simulink model "3_inverse_dynamics_TL"  (R2019b)
settings: Solver=VariableStepAuto  StartTime=0.0  StopTime=2  RelTol=1e-3
undefined symbols (not defined in the file or in its folder): DiscIntNeverNeededParam
libraries: powerlib x4, powerlib_extras x2, simulink x2
settings Model: Creator=liuzhong  LastModifiedBy=李瑾年
settings SFSimCC: CustomCodeUndefinedFunction=UseInterfaceOnly

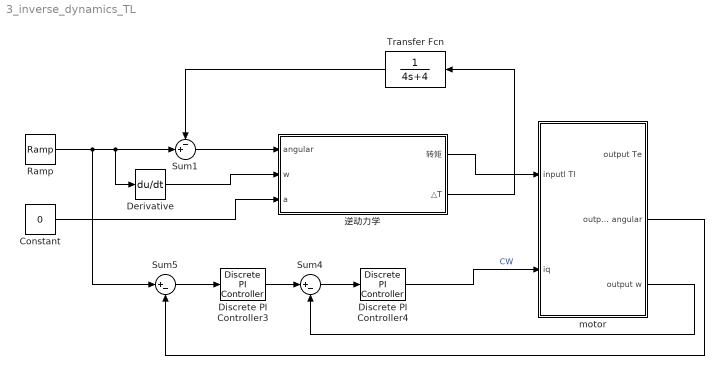
== system 3_inverse_dynamics_TL ==
  Constant : Constant  Value=0
  Derivative : Derivative
  Discrete PI Controller3 : powerlib_extras/Discrete  Control Blocks/Discrete PI Controller  Kp=140  Ki=90  Par_Limits=[1000 -1000]  Init=0  Ts=50e-6
      settings: SourceProductName=Simscape Electrical
  Discrete PI Controller4 : powerlib_extras/Discrete  Control Blocks/Discrete PI Controller  Kp=0.01897  Ki=1.9986  Par_Limits=[300 -300]  Init=0  Ts=50e-6
      settings: SourceProductName=Simscape Electrical
  Ramp : simulink/Sources/Ramp  slope=pi  start=0  InitialOutput=0
  Sum1 : Sum  Inputs=-+|
  Sum4 : Sum  Inputs=|+-
  Sum5 : Sum  Inputs=|+-
  Transfer Fcn : TransferFcn  Denominator=[4 4]
  motor : Subsystem
  逆动力学 : Subsystem
  wires:
  逆动力学/1(转矩) -> motor/1(inputl Tl)
  Sum4/1 -> Discrete PI Controller4/1
  Discrete PI Controller3/1 -> Sum4/1
  Sum5/1 -> Discrete PI Controller3/1
  motor/2(output angular) -> Sum5/2
  motor/3(output w) -> Sum4/2
  Discrete PI Controller4/1 -> motor/2("iq ")  "CW"
  Ramp/1 -> Sum5/1, Sum1/2, Derivative/1
  Derivative/1 -> 逆动力学/2(w)
  Constant/1 -> 逆动力学/3(a)
  逆动力学/2(△T) -> Transfer Fcn/1
  Sum1/1 -> 逆动力学/1("angular ")
  Transfer Fcn/1 -> Sum1/1

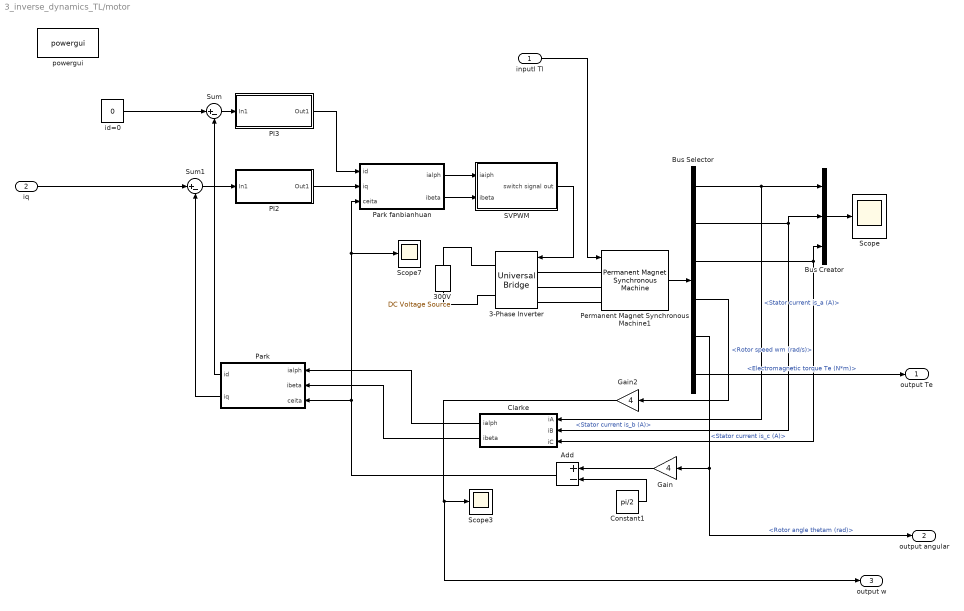
== system 3_inverse_dynamics_TL/motor ==
  inputl Tl : Inport
  "iq " : Inport  Port=2
  3-Phase Inverter : powerlib/Power Electronics/Universal Bridge  Arms=3  SnubberResistance=1e5  SnubberCapacitance=inf  Device=IGBT / Diodes  Ron=1e-3  Lon=0  ForwardVoltages="[  0  0  ]"  ForwardVoltage=0  GTOparameters=[ 10e-6 , 20e-6 ]  IGBTparameters=[ 1e-6 , 2e-6 ]  Measurements=None  Measurements_2=None  converterType=Rectifier
      settings: SourceProductName=Simscape Electrical
  300V : powerlib/Electrical Sources/DC Voltage Source  Amplitude=300  Measurements=Voltage
      settings: SourceProductName=Simscape Electrical
  Add : Sum  Inputs=+-
  Bus Creator : BusCreator  Inputs=3
  Bus Selector : BusSelector  OutputSignals=Stator current is_a (A),Stator current is_b (A),Stator current is_c (A),Rotor speed wm (rad/s),Rotor angle thetam (rad),Electromagnetic torque Te (N*m)
  Clarke : Subsystem
  Constant1 : Constant  Value=pi/2
  Gain : Gain  Gain=4
  Gain2 : Gain  Gain=4
  PI2 : Subsystem
  PI3 : Subsystem
  Park : Subsystem
  Park fanbianhuan : Subsystem
  Permanent Magnet Synchronous Machine1 : powerlib/Machines/Permanent Magnet Synchronous Machine  NbPhases=3  FluxDistribution=Sinusoidal  RotorType=Round  MechanicalLoad=Torque Tm  PresetModel=No  ShowDetailedParameters=on  MeasurementBus=off  Resistance=0.901  Inductance=8.5e-3  dqInductances=[0.02682 0.02682]  La=0.006365  MachineConstant=Torque Constant (N.m / A_peak)  Flux=0.13333  VoltageCst=96.736  TorqueCst=0.8  Flat=120  Mechanical=[0.00012 0.0008 4]  PolePairs=2  InitialConditions=[0,0, 0,0]  InitialConditions5ph=[0 0 0 0 0 0]  RefAngle=90 degrees behind phase A axis (modified Park)  IterativeDiscreteModel=Trapezoidal non iterative  TsBlock=-1  TsPowergui=0
  SVPWM : Subsystem
  Scope : Scope
  Scope3 : Scope
  Scope7 : Scope
  Sum : Sum  Inputs=|+-
  Sum1 : Sum  Inputs=|+-
  id=0 : Constant  Value=0
  powergui : powerlib/powergui  Priority=1  SimulationMode=Discrete  SampleTime=1e-6  frequency=60  Iterations=50  frequencyindice=0  Pbase=100e6  ErrMax=1e-4  UnitsV=kV  UnitsW=MW  buscounter=0  FunctionMessages=off  echomessages=off  EnableUseOfTLC=off  CurrentSourceSwitches=off  DisableSnubberDevices=off  DisableRonSwitches=off  DisableVfSwitches=off  DisplayEquations=off  AutomaticDiscreteSolvers=off  SolverType=Tustin/Backward Euler (TBE)  Interpol=off  ExternalGateDelay=off  methode=off  Ts=100  x0status=blocks  SPID=on  SwTol=0  HookPort=off  NonlinearTolerance=0  nMaxIteration=15  ContinueOnMaxIteration=off  RestoreLinks=warning  ResistiveCurrentMeasurement=off  Frange=[0:2:500]  Ylog=off  Xlog=on  ShowGrid=off  save=off  variable=ZData  structure=0  ZoomFFT=off  StartTime=0.0  cycles=1  DisplayStyle=1  fundamental=60  FreqAxis=off  MaxFrequency=1000  frequencyindicesteady=1  RmsSteady=1  display=off
      settings: SourceProductName=Simscape Electrical
  output Te : Outport  VectorParamsAs1DForOutWhenUnconnected=off
  output angular : Outport  Port=2  VectorParamsAs1DForOutWhenUnconnected=off
  output w : Outport  Port=3  VectorParamsAs1DForOutWhenUnconnected=off
  wires:
  Bus Selector/5 -> output angular/1, Gain/1  "<Rotor angle thetam (rad)>"
  Bus Selector/3 -> Bus Creator/3, Clarke/3(iC)  "<Stator current is_c (A)>"
  Bus Creator/1 -> Scope/1
  Gain/1 -> Add/1
  Bus Selector/2 -> Bus Creator/2, Clarke/2(iB)  "<Stator current is_b (A)>"
  Bus Selector/4 -> Gain2/1  "<Rotor speed wm (rad/s)>"
  Park fanbianhuan/2("ibeta ") -> SVPWM/2(ibeta)
  Sum/1 -> PI3/1(In1)
  Park/1(id) -> Sum/2
  Clarke/1(ialph) -> Park/1(ialph)
  Bus Selector/6 -> output Te/1  "<Electromagnetic torque Te (N*m)>"
  id=0/1 -> Sum/1
  SVPWM/1(switch signal out) -> 3-Phase Inverter/1
  Park/2(iq) -> Sum1/2
  PI3/1(Out1) -> Park fanbianhuan/1(id)
  Park fanbianhuan/1(ialph) -> SVPWM/1(iaiph)
  Add/1 -> Scope7/1, Park fanbianhuan/3(ceita), Park/3(ceita)
  Clarke/2(ibeta) -> Park/2(ibeta)
  Sum1/1 -> PI2/1(In1)
  PI2/1(Out1) -> Park fanbianhuan/2(iq)
  inputl Tl/1 -> Permanent Magnet Synchronous Machine1/1
  Constant1/1 -> Add/2
  "iq "/1 -> Sum1/1
  Permanent Magnet Synchronous Machine1/1 -> Bus Selector/1
  Bus Selector/1 -> Bus Creator/1, Clarke/1(iA)  "<Stator current is_a (A)>"
  Gain2/1 -> output w/1, Scope3/1
  connections:
  Permanent Magnet Synchronous Machine1/LConn1 -- 3-Phase Inverter/LConn1
  Permanent Magnet Synchronous Machine1/LConn3 -- 3-Phase Inverter/LConn3
  300V/RConn1 -- 3-Phase Inverter/RConn1
  3-Phase Inverter/RConn2 -- 300V/LConn1
  Permanent Magnet Synchronous Machine1/LConn2 -- 3-Phase Inverter/LConn2

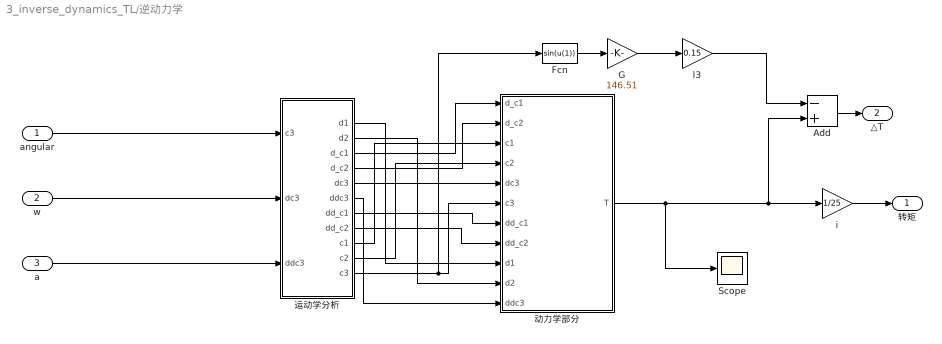
== system 3_inverse_dynamics_TL/逆动力学 ==
  "angular " : Inport
  w : Inport  Port=2
  a : Inport  Port=3
  Add : Sum  Inputs=-+
  Fcn : Fcn  Expr=sin(u(1))
  G : Gain  Gain=146.51
  Scope : Scope
  i : Gain  Gain=1/25
  l3 : Gain  Gain=0.15
  动力学部分 : Subsystem
  运动学分析 : Subsystem
  转矩 : Outport  VectorParamsAs1DForOutWhenUnconnected=off
  △T : Outport  Port=2  VectorParamsAs1DForOutWhenUnconnected=off
  wires:
  运动学分析/6(ddc3) -> 动力学部分/11(ddc3)
  运动学分析/5(dc3) -> 动力学部分/5(dc3)
  动力学部分/1(T) -> Scope/1, Add/2, i/1
  运动学分析/4(d_c2) -> 动力学部分/2(d_c2)
  运动学分析/3(d_c1) -> 动力学部分/1(d_c1)
  运动学分析/11("c3 ") -> Fcn/1, 动力学部分/6(c3)
  运动学分析/10("c2 ") -> 动力学部分/4(c2)
  运动学分析/9("c1 ") -> 动力学部分/3(c1)
  运动学分析/8(dd_c2) -> 动力学部分/8(dd_c2)
  运动学分析/7(dd_c1) -> 动力学部分/7(dd_c1)
  运动学分析/2(d2) -> 动力学部分/10(d2)
  运动学分析/1(d1) -> 动力学部分/9(d1)
  "angular "/1 -> 运动学分析/1(c3)
  Add/1 -> △T/1
  Fcn/1 -> G/1
  G/1 -> l3/1
  l3/1 -> Add/1
  w/1 -> 运动学分析/2("dc3  ")
  a/1 -> 运动学分析/3("ddc3 ")
  i/1 -> 转矩/1

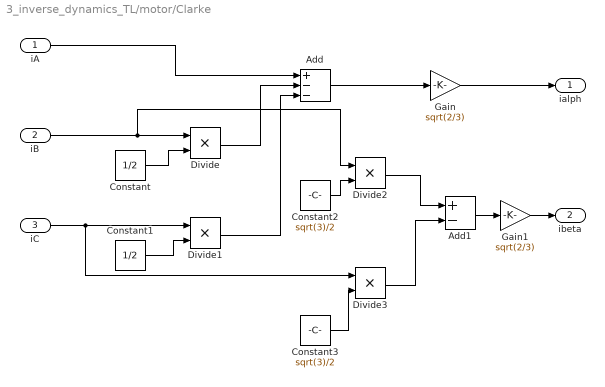
== system 3_inverse_dynamics_TL/motor/Clarke ==
  iA : Inport
  iB : Inport  Port=2
  iC : Inport  Port=3
  Add : Sum  Inputs=+--
  Add1 : Sum  Inputs=+-
  Constant : Constant  Value=1/2
  Constant1 : Constant  Value=1/2
  Constant2 : Constant  Value=sqrt(3)/2
  Constant3 : Constant  Value=sqrt(3)/2
  Divide{,1..3} (4 alike) : Product  Inputs=**
  Gain : Gain  Gain=sqrt(2/3)
  Gain1 : Gain  Gain=sqrt(2/3)
  ialph : Outport  VectorParamsAs1DForOutWhenUnconnected=off
  ibeta : Outport  Port=2  VectorParamsAs1DForOutWhenUnconnected=off
  wires:
  Add/1 -> Gain/1
  iA/1 -> Add/1
  iB/1 -> Divide/1, Divide2/1
  Constant/1 -> Divide/2
  Divide/1 -> Add/2
  iC/1 -> Divide1/1, Divide3/1
  Constant1/1 -> Divide1/2
  Divide1/1 -> Add/3
  Constant2/1 -> Divide2/2
  Divide2/1 -> Add1/1
  Constant3/1 -> Divide3/2
  Divide3/1 -> Add1/2
  Add1/1 -> Gain1/1
  Gain/1 -> ialph/1
  Gain1/1 -> ibeta/1

== system 3_inverse_dynamics_TL/motor/PI2 ==
  In1 : Inport
  Add : Sum
  Discrete-Time Integrator : DiscreteIntegrator  SampleTime=50e-6  LimitOutput=on  UpperSaturationLimit=500  LowerSaturationLimit=-500  ICPrevOutput=DiscIntNeverNeededParam  ICPrevScaledInput=DiscIntNeverNeededParam
  Ki : Gain  Gain=7700
  Kp : Gain  Gain=50
  Saturation : Saturate  UpperLimit=300  LowerLimit=-300
  Zero-Order Hold : ZeroOrderHold  SampleTime=50e-6
  Out1 : Outport  VectorParamsAs1DForOutWhenUnconnected=off
  wires:
  Kp/1 -> Zero-Order Hold/1
  Ki/1 -> Discrete-Time Integrator/1
  In1/1 -> Ki/1, Kp/1
  Zero-Order Hold/1 -> Add/1
  Discrete-Time Integrator/1 -> Add/2
  Add/1 -> Saturation/1
  Saturation/1 -> Out1/1

== system 3_inverse_dynamics_TL/motor/PI3 ==
  In1 : Inport
  Add : Sum
  Discrete-Time Integrator : DiscreteIntegrator  SampleTime=50e-6  LimitOutput=on  UpperSaturationLimit=500  LowerSaturationLimit=-500  ICPrevOutput=DiscIntNeverNeededParam  ICPrevScaledInput=DiscIntNeverNeededParam
  Ki : Gain  Gain=7700
  Kp : Gain  Gain=50
  Saturation : Saturate  UpperLimit=300  LowerLimit=-300
  Zero-Order Hold : ZeroOrderHold  SampleTime=50e-6
  Out1 : Outport  VectorParamsAs1DForOutWhenUnconnected=off
  wires:
  Kp/1 -> Zero-Order Hold/1
  Ki/1 -> Discrete-Time Integrator/1
  In1/1 -> Ki/1, Kp/1
  Zero-Order Hold/1 -> Add/1
  Discrete-Time Integrator/1 -> Add/2
  Add/1 -> Saturation/1
  Saturation/1 -> Out1/1

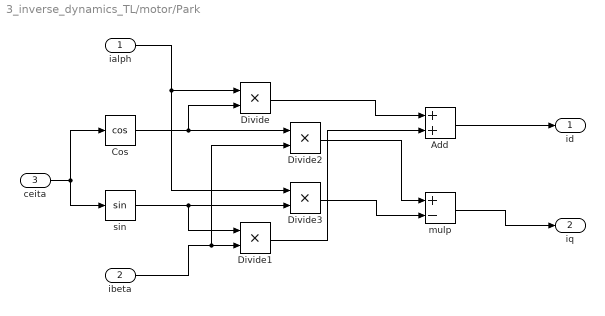
== system 3_inverse_dynamics_TL/motor/Park ==
  ialph : Inport
  ibeta : Inport  Port=2
  ceita : Inport  Port=3
  Add : Sum
  Cos : Trigonometry  Operator=cos
  Divide{,1..3} (4 alike) : Product  Inputs=**
  mulp : Sum  Inputs=+-
  sin : Trigonometry
  id : Outport  VectorParamsAs1DForOutWhenUnconnected=off
  iq : Outport  Port=2  VectorParamsAs1DForOutWhenUnconnected=off
  wires:
  ceita/1 -> sin/1, Cos/1
  ialph/1 -> Divide/1, Divide3/1
  Cos/1 -> Divide2/1, Divide/2
  sin/1 -> Divide1/1, Divide3/2
  ibeta/1 -> Divide2/2, Divide1/2
  Divide/1 -> Add/1
  Divide1/1 -> Add/2
  Add/1 -> id/1
  Divide2/1 -> mulp/1
  Divide3/1 -> mulp/2
  mulp/1 -> iq/1

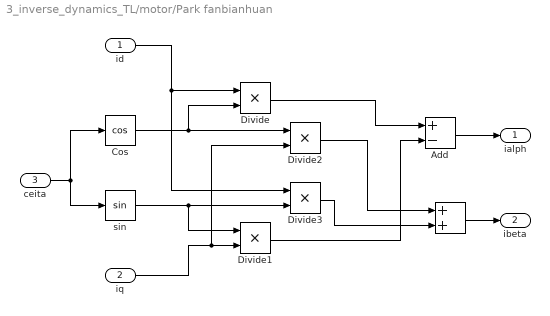
== system 3_inverse_dynamics_TL/motor/Park fanbianhuan ==
  id : Inport
  iq : Inport  Port=2
  ceita : Inport  Port=3
  " " : Sum
  Add : Sum  Inputs=+-
  Cos : Trigonometry  Operator=cos
  Divide{,1..3} (4 alike) : Product  Inputs=**
  sin : Trigonometry
  ialph : Outport  VectorParamsAs1DForOutWhenUnconnected=off
  "ibeta " : Outport  Port=2  VectorParamsAs1DForOutWhenUnconnected=off
  wires:
  ceita/1 -> sin/1, Cos/1
  id/1 -> Divide/1, Divide3/1
  Cos/1 -> Divide2/1, Divide/2
  sin/1 -> Divide1/1, Divide3/2
  iq/1 -> Divide2/2, Divide1/2
  Divide/1 -> Add/1
  Divide1/1 -> Add/2
  Add/1 -> ialph/1
  Divide2/1 -> " "/1
  Divide3/1 -> " "/2
  " "/1 -> "ibeta "/1

== system 3_inverse_dynamics_TL/motor/SVPWM ==
  iaiph : Inport
  ibeta : Inport  Port=2
  compute time : Subsystem
  "select location " : Subsystem
  switch signal : Subsystem
  switch signal out : Outport  VectorParamsAs1DForOutWhenUnconnected=off
  wires:
  iaiph/1 -> compute time/2(Ualph), "select location "/1(Uaiph)
  ibeta/1 -> "select location "/2(Ubeta), compute time/3(Ubeta)
  "select location "/1(location) -> compute time/1(location), switch signal/1(location)
  compute time/1(t1) -> switch signal/2(T1)
  compute time/2(t2) -> switch signal/3(T2)
  compute time/3(t0) -> switch signal/4(T0)
  switch signal/1(signal) -> switch signal out/1

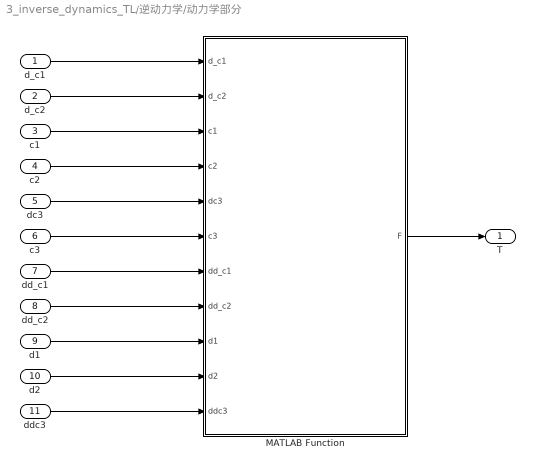
== system 3_inverse_dynamics_TL/逆动力学/动力学部分 ==
  d_c1 : Inport
  d_c2 : Inport  Port=2
  c1 : Inport  Port=3
  c2 : Inport  Port=4
  dc3 : Inport  Port=5
  c3 : Inport  Port=6
  dd_c1 : Inport  Port=7
  dd_c2 : Inport  Port=8
  d1 : Inport  Port=9
  d2 : Inport  Port=10
  ddc3 : Inport  Port=11
  MATLAB Function : MATLAB Function  TreatAsAtomicUnit=on
  T : Outport  VectorParamsAs1DForOutWhenUnconnected=off
  wires:
  d_c1/1 -> MATLAB Function/1(d_c1)
  d_c2/1 -> MATLAB Function/2(d_c2)
  c1/1 -> MATLAB Function/3(c1)
  c2/1 -> MATLAB Function/4(c2)
  dc3/1 -> MATLAB Function/5(dc3)
  c3/1 -> MATLAB Function/6(c3)
  dd_c1/1 -> MATLAB Function/7(dd_c1)
  dd_c2/1 -> MATLAB Function/8(dd_c2)
  d1/1 -> MATLAB Function/9(d1)
  d2/1 -> MATLAB Function/10(d2)
  ddc3/1 -> MATLAB Function/11(ddc3)
  MATLAB Function/1(F) -> T/1

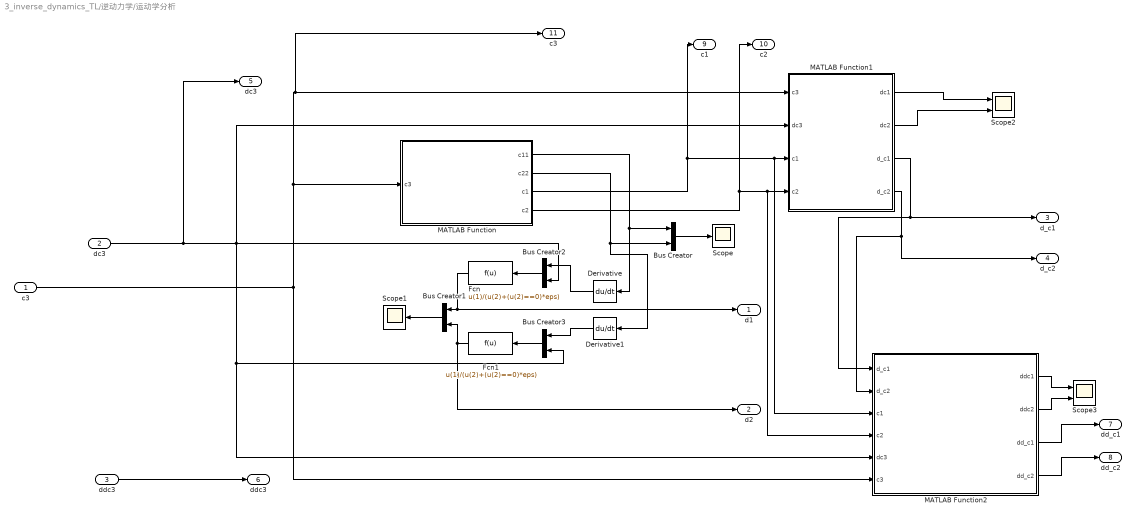
== system 3_inverse_dynamics_TL/逆动力学/运动学分析 ==
  c3 : Inport
  "dc3  " : Inport  Port=2
  "ddc3 " : Inport  Port=3
  Bus Creator{,1..3} (4 alike) : BusCreator  Inputs=2
  Derivative : Derivative
  Derivative1 : Derivative
  Fcn : Fcn  Expr=u(1)/(u(2)+(u(2)==0)*eps)
  Fcn1 : Fcn  Expr=u(1)/(u(2)+(u(2)==0)*eps)
  MATLAB Function : MATLAB Function  TreatAsAtomicUnit=on
  MATLAB Function1 : MATLAB Function  TreatAsAtomicUnit=on
  MATLAB Function2 : MATLAB Function  TreatAsAtomicUnit=on
  Scope : Scope
  Scope1 : Scope
  Scope2 : Scope  NumInputPorts=2
  Scope3 : Scope  NumInputPorts=2
  d1 : Outport  VectorParamsAs1DForOutWhenUnconnected=off
  d2 : Outport  Port=2  VectorParamsAs1DForOutWhenUnconnected=off
  d_c1 : Outport  Port=3  VectorParamsAs1DForOutWhenUnconnected=off
  d_c2 : Outport  Port=4  VectorParamsAs1DForOutWhenUnconnected=off
  dc3 : Outport  Port=5  VectorParamsAs1DForOutWhenUnconnected=off
  ddc3 : Outport  Port=6  VectorParamsAs1DForOutWhenUnconnected=off
  dd_c1 : Outport  Port=7  VectorParamsAs1DForOutWhenUnconnected=off
  dd_c2 : Outport  Port=8  VectorParamsAs1DForOutWhenUnconnected=off
  "c1 " : Outport  Port=9  VectorParamsAs1DForOutWhenUnconnected=off
  "c2 " : Outport  Port=10  VectorParamsAs1DForOutWhenUnconnected=off
  "c3 " : Outport  Port=11  VectorParamsAs1DForOutWhenUnconnected=off
  wires:
  MATLAB Function/1(c11) -> Derivative/1, Bus Creator/1
  MATLAB Function/2(c22) -> Derivative1/1, Bus Creator/2
  Bus Creator1/1 -> Scope1/1
  c3/1 -> "c3 "/1, MATLAB Function1/1(c3), MATLAB Function/1(c3), MATLAB Function2/6(c3)
  Bus Creator/1 -> Scope/1
  Bus Creator2/1 -> Fcn/1
  Derivative/1 -> Bus Creator2/1
  Fcn/1 -> d1/1, Bus Creator1/1
  Fcn1/1 -> d2/1, Bus Creator1/2
  Bus Creator3/1 -> Fcn1/1
  Derivative1/1 -> Bus Creator3/1
  MATLAB Function/3(c1) -> "c1 "/1, MATLAB Function2/3(c1), MATLAB Function1/3(c1)
  MATLAB Function/4(c2) -> "c2 "/1, MATLAB Function2/4(c2), MATLAB Function1/4(c2)
  MATLAB Function1/3(d_c1) -> d_c1/1, MATLAB Function2/1(d_c1)
  MATLAB Function1/4(d_c2) -> MATLAB Function2/2(d_c2), d_c2/1
  MATLAB Function2/4(dd_c2) -> dd_c2/1
  MATLAB Function2/3(dd_c1) -> dd_c1/1
  MATLAB Function1/1(dc1) -> Scope2/1
  MATLAB Function1/2(dc2) -> Scope2/2
  MATLAB Function2/1(ddc1) -> Scope3/1
  MATLAB Function2/2(ddc2) -> Scope3/2
  "dc3  "/1 -> dc3/1, MATLAB Function1/2(dc3), Bus Creator2/2, Bus Creator3/2, MATLAB Function2/5(dc3)
  "ddc3 "/1 -> ddc3/1

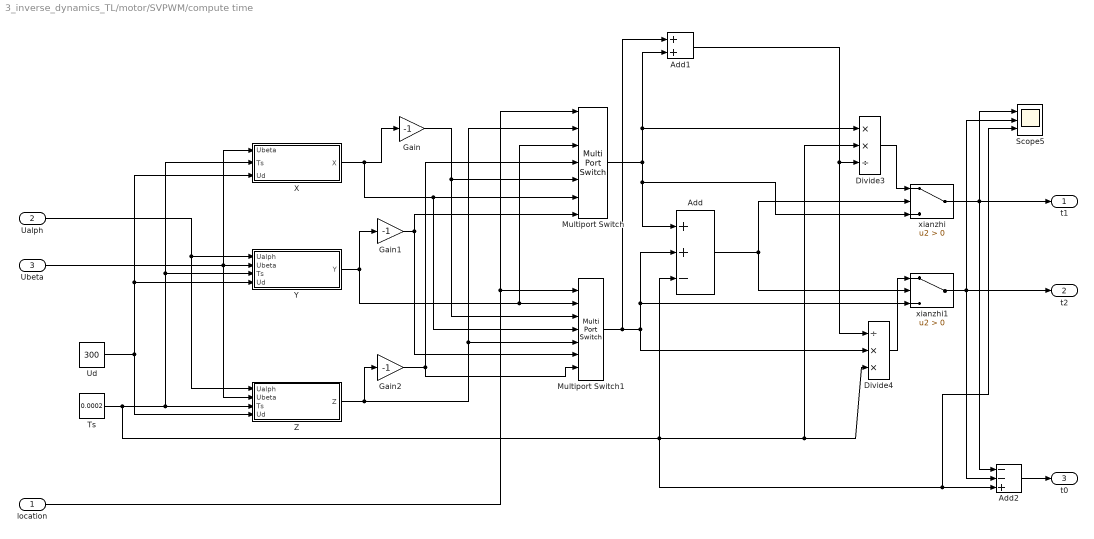
== system 3_inverse_dynamics_TL/motor/SVPWM/compute time ==
  location : Inport
  Ualph : Inport  Port=2
  Ubeta : Inport  Port=3
  Add : Sum  Inputs=++-
  Add1 : Sum
  Add2 : Sum  Inputs=--+
  Divide3 : Product  Inputs=**/
  Divide4 : Product  Inputs=/**
  Gain : Gain  Gain=-1
  Gain1 : Gain  Gain=-1
  Gain2 : Gain  Gain=-1
  Multiport Switch : MultiPortSwitch  Inputs=6  DiagnosticForDefault=None
  Multiport Switch1 : MultiPortSwitch  Inputs=6  DiagnosticForDefault=None
  Scope5 : Scope  NumInputPorts=3
  Ts : Constant  Value=0.0002
  Ud : Constant  Value=300
  X : Subsystem
  Y : Subsystem
  Z : Subsystem
  xianzhi : Switch  Criteria=u2 > Threshold
  xianzhi1 : Switch  Criteria=u2 > Threshold
  t1 : Outport  VectorParamsAs1DForOutWhenUnconnected=off
  t2 : Outport  Port=2  VectorParamsAs1DForOutWhenUnconnected=off
  t0 : Outport  Port=3  VectorParamsAs1DForOutWhenUnconnected=off
  wires:
  Ualph/1 -> Y/1(Ualph), Z/1(Ualph)
  Ubeta/1 -> X/1(Ubeta), Y/2(Ubeta), Z/2(Ubeta)
  Ts/1 -> Add/3, Divide3/2, Divide4/3, Scope5/3, Add2/3, X/2(Ts), Y/3(Ts), Z/3(Ts)
  Ud/1 -> Z/4(Ud), X/3(Ud), Y/4(Ud)
  Y/1(Y) -> Gain1/1, Multiport Switch/3, Multiport Switch1/2
  Z/1(Z) -> Gain2/1, Multiport Switch1/5, Multiport Switch/2
  Gain/1 -> Multiport Switch1/3, Multiport Switch/5
  Gain2/1 -> Multiport Switch1/7, Multiport Switch/4
  X/1(X) -> Gain/1, Multiport Switch1/4, Multiport Switch/6
  Gain1/1 -> Multiport Switch/7, Multiport Switch1/6
  Add/1 -> xianzhi1/2, xianzhi/2
  Multiport Switch/1 -> Divide3/1, Add1/2, xianzhi/3, Add/1
  Multiport Switch1/1 -> Add1/1, Divide4/2, Add/2, xianzhi1/3
  xianzhi/1 -> Scope5/1, Add2/1, t1/1
  xianzhi1/1 -> Scope5/2, Add2/2, t2/1
  Add1/1 -> Divide3/3, Divide4/1
  Divide3/1 -> xianzhi/1
  Divide4/1 -> xianzhi1/1
  location/1 -> Multiport Switch/1, Multiport Switch1/1
  Add2/1 -> t0/1

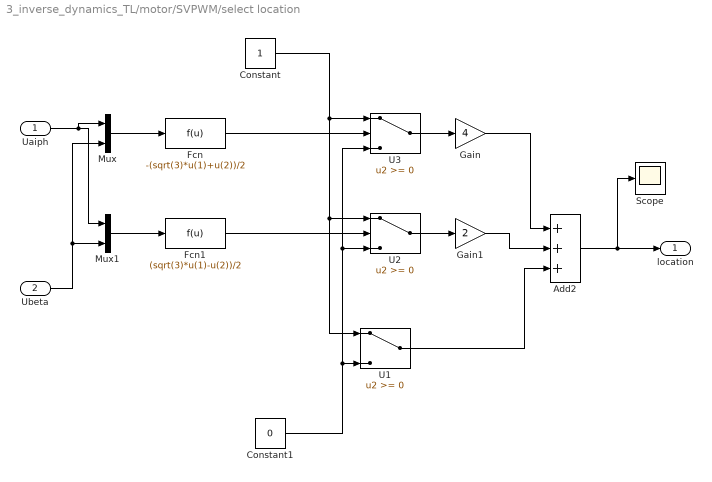
== system 3_inverse_dynamics_TL/motor/SVPWM/select location  ==
  Uaiph : Inport
  Ubeta : Inport  Port=2
  Add2 : Sum  Inputs=+++
  Constant : Constant
  Constant1 : Constant  Value=0
  Fcn : Fcn  Expr=-(sqrt(3)*u(1)+u(2))/2
  Fcn1 : Fcn  Expr=(sqrt(3)*u(1)-u(2))/2
  Gain : Gain  Gain=4
  Gain1 : Gain  Gain=2
  Mux : Mux  Inputs=2
  Mux1 : Mux  Inputs=2
  Scope : Scope
  U1 : Switch
  U2 : Switch
  U3 : Switch
  location : Outport  VectorParamsAs1DForOutWhenUnconnected=off
  wires:
  Constant1/1 -> U1/3, U2/3, U3/3
  Constant/1 -> U3/1, U2/1, U1/1
  Fcn/1 -> U3/2
  Fcn1/1 -> U2/2
  U2/1 -> Gain1/1
  U1/1 -> Add2/3
  Gain/1 -> Add2/1
  Gain1/1 -> Add2/2
  Add2/1 -> Scope/1, location/1
  U3/1 -> Gain/1
  Uaiph/1 -> Mux1/1, Mux/1
  Mux/1 -> Fcn/1
  Ubeta/1 -> Mux1/2, Mux/2
  Mux1/1 -> Fcn1/1

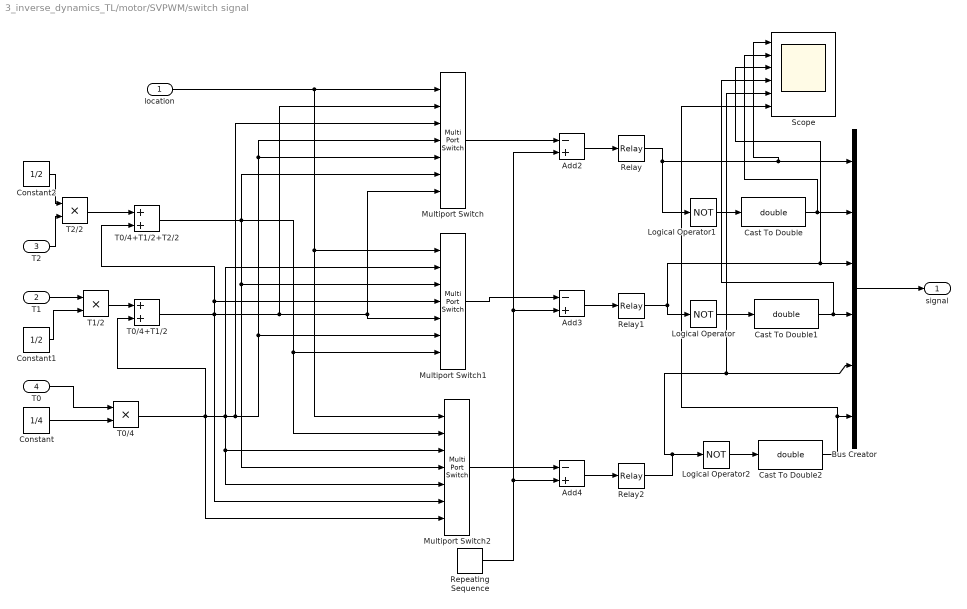
== system 3_inverse_dynamics_TL/motor/SVPWM/switch signal ==
  location : Inport
  T1 : Inport  Port=2
  T2 : Inport  Port=3
  T0 : Inport  Port=4
  Add2 : Sum  Inputs=-+
  Add3 : Sum  Inputs=-+
  Add4 : Sum  Inputs=-+
  Bus Creator : BusCreator  Inputs=6
  Cast To Double : DataTypeConversion  OutDataTypeStr=double
  Cast To Double1 : DataTypeConversion  OutDataTypeStr=double
  Cast To Double2 : DataTypeConversion  OutDataTypeStr=double
  Constant : Constant  Value=1/4
  Constant1 : Constant  Value=1/2
  Constant2 : Constant  Value=1/2
  Logical Operator : Logic  Operator=NOT  AllPortsSameDT=off  OutDataTypeStr=boolean
  Logical Operator1 : Logic  Operator=NOT  AllPortsSameDT=off  OutDataTypeStr=boolean
  Logical Operator2 : Logic  Operator=NOT  AllPortsSameDT=off  OutDataTypeStr=boolean
  Multiport Switch : MultiPortSwitch  Inputs=6  DiagnosticForDefault=None
  Multiport Switch1 : MultiPortSwitch  Inputs=6  DiagnosticForDefault=None
  Multiport Switch2 : MultiPortSwitch  Inputs=6  DiagnosticForDefault=None
  Relay : Relay
  Relay1 : Relay
  Relay2 : Relay
  Repeating Sequence : simulink/Sources/Repeating Sequence  rep_seq_t=[0 0.0001 0.0002]  rep_seq_y=[0 0.0001 0]
  Scope : Scope  NumInputPorts=6
  T0/4 : Product  Inputs=**
  T0/4+T1/2 : Sum
  T0/4+T1/2+T2/2 : Sum
  T1/2 : Product  Inputs=**
  T2/2 : Product  Inputs=**
  signal : Outport  VectorParamsAs1DForOutWhenUnconnected=off
  wires:
  location/1 -> Multiport Switch/1, Multiport Switch1/1, Multiport Switch2/1
  Constant/1 -> T0/4/2
  T0/1 -> T0/4/1
  T0/4/1 -> Multiport Switch2/5, Multiport Switch2/3, Multiport Switch/3, Multiport Switch/4, Multiport Switch/5, Multiport Switch1/6, Multiport Switch1/2, Multiport Switch2/7, T0/4+T1/2/2
  T2/1 -> T2/2/2
  T0/4+T1/2/1 -> Multiport Switch1/5, Multiport Switch/7, Multiport Switch/2, T0/4+T1/2+T2/2/2, Multiport Switch1/4, Multiport Switch2/6
  Multiport Switch/1 -> Add2/1
  Multiport Switch1/1 -> Add3/1
  Multiport Switch2/1 -> Add4/1
  T1/2/1 -> T0/4+T1/2/1
  T1/1 -> T1/2/1
  Constant1/1 -> T1/2/2
  Constant2/1 -> T2/2/1
  T2/2/1 -> T0/4+T1/2+T2/2/1
  Repeating Sequence/1 -> Add3/2, Add2/2, Add4/2
  Add2/1 -> Relay/1
  Add4/1 -> Relay2/1
  Add3/1 -> Relay1/1
  Relay1/1 -> Logical Operator/1, Scope/3, Bus Creator/3
  Relay/1 -> Logical Operator1/1, Scope/1, Bus Creator/1
  Logical Operator1/1 -> Cast To Double/1
  Relay2/1 -> Bus Creator/5, Scope/5, Logical Operator2/1
  Bus Creator/1 -> signal/1
  Logical Operator/1 -> Cast To Double1/1
  Cast To Double/1 -> Scope/2, Bus Creator/2
  Cast To Double1/1 -> Scope/4, Bus Creator/4
  Cast To Double2/1 -> Scope/6, Bus Creator/6
  Logical Operator2/1 -> Cast To Double2/1
  T0/4+T1/2+T2/2/1 -> Multiport Switch1/3, Multiport Switch2/4, Multiport Switch/6, Multiport Switch1/7, Multiport Switch2/2

== system 3_inverse_dynamics_TL/motor/SVPWM/compute time/X ==
  Ubeta : Inport
  Ts : Inport  Port=2
  Ud : Inport  Port=3
  Constant1 : Constant  Value=sqrt(3)
  Divide : Product  Inputs=**
  Divide1 : Product  Inputs=**/
  X : Outport  VectorParamsAs1DForOutWhenUnconnected=off
  wires:
  Ubeta/1 -> Divide/1
  Constant1/1 -> Divide/2
  Divide/1 -> Divide1/1
  Ts/1 -> Divide1/2
  Ud/1 -> Divide1/3
  Divide1/1 -> X/1

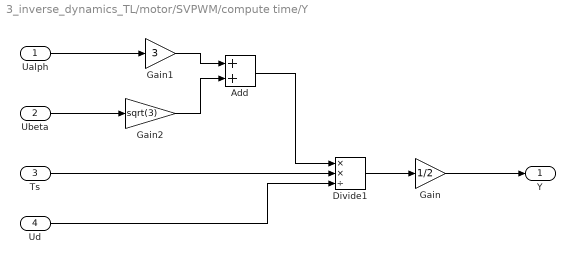
== system 3_inverse_dynamics_TL/motor/SVPWM/compute time/Y ==
  Ualph : Inport
  Ubeta : Inport  Port=2
  Ts : Inport  Port=3
  Ud : Inport  Port=4
  Add : Sum
  Divide1 : Product  Inputs=**/
  Gain : Gain  Gain=1/2
  Gain1 : Gain  Gain=3
  Gain2 : Gain  Gain=sqrt(3)
  Y : Outport  VectorParamsAs1DForOutWhenUnconnected=off
  wires:
  Ud/1 -> Divide1/3
  Ts/1 -> Divide1/2
  Divide1/1 -> Gain/1
  Ubeta/1 -> Gain2/1
  Ualph/1 -> Gain1/1
  Gain1/1 -> Add/1
  Gain2/1 -> Add/2
  Add/1 -> Divide1/1
  Gain/1 -> Y/1

== system 3_inverse_dynamics_TL/motor/SVPWM/compute time/Z ==
  Ualph : Inport
  Ubeta : Inport  Port=2
  Ts : Inport  Port=3
  Ud : Inport  Port=4
  Add : Sum  Inputs=-+
  Divide1 : Product  Inputs=**/
  Gain : Gain  Gain=1/2
  Gain1 : Gain  Gain=3
  Gain2 : Gain  Gain=sqrt(3)
  Z : Outport  VectorParamsAs1DForOutWhenUnconnected=off
  wires:
  Gain2/1 -> Add/2
  Add/1 -> Divide1/1
  Ualph/1 -> Gain1/1
  Ud/1 -> Divide1/3
  Gain/1 -> Z/1
  Divide1/1 -> Gain/1
  Ts/1 -> Divide1/2
  Gain1/1 -> Add/1
  Ubeta/1 -> Gain2/1

== matlab function 3_inverse_dynamics_TL/逆动力学/运动学分析/MATLAB Function ==
  settings: sampleTime=1e-5
  data: c3 input; c11 output; c22 output; c1 output; c2 output
function [c11,c22,c1,c2] = prantice_angle(c3)
%=====================已知参数==================================%
a=0.5;%髋关节到曲柄中心间垂直距离
ceta4=0.499;%髋关节到曲柄中心连线与水平面间的角度
l1=0.44;%大腿简化长度
l2=0.390;%小腿简化长度
l3=0.150;%脚简化长度
l4=a./sin(ceta4);%髋关节到曲柄中心连线距离
m1=9.843;%大腿质量
m2=3.626;%小腿质量
m3=1.182;%脚质量
I1=12.23;I2=3.14;I3=2.569;%大腿、小腿和脚在水平面内（绕z轴）转动惯量
g=10;%垂直加速度
%================================================================%
A1=l4.*cos(ceta4)+l3.*cos(c3);
A2=l4.*sin(ceta4)+l3.*sin(c3);
A3=(l1.^2+A1.^2+A2.^2-l2.^2)./(2.*l1);
%c1=2.*atan((A2+(A1.^2+A2.^2-A3.^2).^(0.5))./(A1+A3));%c1表示角ceta1
c1=2.*atan((A2+sqrt(complex((A1.^2+A2.^2-A3.^2))))./(A1+A3));%c1表示角ceta1
c2=atan((l4.*sin(ceta4)+l3.*sin(c3)-l1.*sin(c1))./(l4.*cos(ceta4)+l3.*cos(c3)-l1*cos(c1)));%c2表示角ceta2
c11=abs(c1);
c22=abs(c2);
%dc1dc3=diff(c11,c3);
%dc2dc3=diff(c22,c3);
%d1=abs(dc1dc3);
%d2=abs(dc2dc3);

== matlab function 3_inverse_dynamics_TL/逆动力学/运动学分析/MATLAB Function1 ==
  data: c3 input; dc1 output; dc3 input; c1 input; c2 input; dc2 output; d_c1 output; d_c2 output
function [dc1,dc2,d_c1,d_c2] = practice_angular_speed(c3,dc3,c1,c2)
%=====================已知参数==================================%
a=0.5;%髋关节到曲柄中心间垂直距离
ceta4=0.499;%髋关节到曲柄中心连线与水平面间的角度
l1=0.44;%大腿简化长度
l2=0.390;%小腿简化长度
l3=0.150;%脚简化长度
l4=a./sin(ceta4);%髋关节到曲柄中心连线距离
m1=9.843;%大腿质量
m2=3.626;%小腿质量
m3=1.182;%脚质量
I1=12.23;I2=3.14;I3=2.569;%大腿、小腿和脚在水平面内（绕z轴）转动惯量
g=10;%垂直加速度
%================================================================%
d_c1=l3.*sin(c2-c3)./(l1.*sin(c2-c1));
d_c2=l3.*sin(c3-c1)./(l2.*sin(c2-c1));
dc1=d_c1;
dc2=d_c2;

== matlab function 3_inverse_dynamics_TL/逆动力学/运动学分析/MATLAB Function2 ==
  data: d_c1 input; ddc1 output; d_c2 input; c1 input; c2 input; dc3 input; c3 input; ddc2 output; dd_c1 output; dd_c2 output
function [ddc1,ddc2,dd_c1,dd_c2] = practice_angular_acceleration(d_c1,d_c2,c1,c2,dc3,c3)
%=====================已知参数==================================%
a=0.5;%髋关节到曲柄中心间垂直距离
ceta4=0.499;%髋关节到曲柄中心连线与水平面间的角度
l1=0.44;%大腿简化长度
l2=0.390;%小腿简化长度
l3=0.150;%脚简化长度
l4=a./sin(ceta4);%髋关节到曲柄中心连线距离
m1=9.843;%大腿质量
m2=3.626;%小腿质量
m3=1.182;%脚质量
I1=12.23;I2=3.14;I3=2.569;%大腿、小腿和脚在水平面内（绕z轴）转动惯量
g=10;%垂直加速度
%================================================================%
B1=dc3.^2.*(-l3.*sin(c3))-(-l1.*sin(c1).*d_c1.^2-l2.*sin(c2).*d_c2.^2)
B2=dc3.^2.*(l3.*cos(c3))-(l1.*cos(c1).*d_c1.^2+l2.*cos(c2).*d_c2.^2);
dd_c1=(-B1.*l2.*sin(c2)-B2.*l2.*cos(c2))./(l1.*l2.*sin(c1-c2));
dd_c2=(B1.*l1.*sin(c1)+B2.*l1.*cos(c1))./(l1.*l2.*sin(c1-c2));
ddc1=abs(dd_c1);
ddc2=abs(dd_c2);

== matlab function 3_inverse_dynamics_TL/逆动力学/动力学部分/MATLAB Function ==
  data: d_c1 input; F output; d_c2 input; c1 input; c2 input; dc3 input; c3 input; dd_c1 input; dd_c2 input; d1 input; d2 input; ddc3 input
function F  = fcn(d_c1,d_c2,c1,c2,dc3,c3,dd_c1,dd_c2,d1,d2,ddc3)
%=====================已知参数==================================%
a=0.5;%髋关节到曲柄中心间垂直距离
ceta4=0.499;%髋关节到曲柄中心连线与水平面间的角度
l1=0.44;%大腿简化长度
l2=0.390;%小腿简化长度
l3=0.150;%脚简化长度
l4=a./sin(ceta4);%髋关节到曲柄中心连线距离
m1=9.843;%大腿质量
m2=3.626;%小腿质量
m3=1.182;%脚质量
I1=12.23;I2=3.14;I3=2.569;%大腿、小腿和脚在水平面内（绕z轴）转动惯量
g=10;%垂直加速度
%================================================================%
P1=l3.*sin(c2-c3)./(l1.*sin(c2-c1));
b1=l3./l1.*((cos(c2-c3)./sin(c2-c1).*(dc3.*d2-dc3))-((cos(c2-c1).*sin(c2-c3))./(sin(c2-c1).^2).*(dc3.*(d2-d1))));
a1=(1/4.*m1.*l1.^2).*((ddc3.*P1+dc3.*b1).*P1+b1.*d_c1);

P2=l3.*sin(c3-c1)./(l2.*sin(c2-c1));
b2=l3./l2.*((cos(c3-c1)./sin(c2-c1).*(dc3-d2.*dc3))-((cos(c2-c1).*sin(c3-c1))./(sin(c2-c1).^2).*(dc3.*(d2-d1))));
a2=(1/4.*m2.*l2.^2).*((ddc3.*P2+dc3.*b2).*P2+d_c2.*b2);

a3=1/4.*(m3.*l3.^2+I3).*ddc3;
a4=a1+a2+a3;
%============================拉格朗日方程的第一部分：动能想对于广义坐标的微分========================================%
b5=l3./l1.*((cos(c2-c3)./sin(c2-c1).*(d2-1))-(cos(c2-c1)./(sin(c2-c1).^2).*sin(c2-c3).*(d2-d1)));
a5=(1/4.*m1.*l1.^2+I1).*d_c1.*dc3.*b5;

b6=l3./l2.*((cos(c3-c1)./sin(c2-c1).*(1-d1))-(cos(c2-c1)./(sin(c2-c1).^2).*sin(c3-c1).*(d2-d1)));
a6=(1/4.*m2.*l2.^2+I2).*d_c2.*dc3.*b6;

a7=m1.*g.*(a+l1.*cos(c1)./2.*d1);
a8=m2.*g.*(a+l1.*cos(c1).*d1-l2.*cos(c2).*d2./2);
a9=1/2.*m3.*g.*l3.*cos(c3);
a10=a5+a6-a7-a8-a9;
f=a4-a10;
F=abs(f);

%============================拉格朗日方程的第一部分：势能想对于广义坐标的微分========================================%
